simulink model "robot_forward"  (R2017a)
settings: Solver=FixedStepAuto  StartTime=0.0  StopTime=20  FixedStep=1e-3  RelTol=1e-3
settings Model: Creator=Jan  LastModifiedBy=Jan

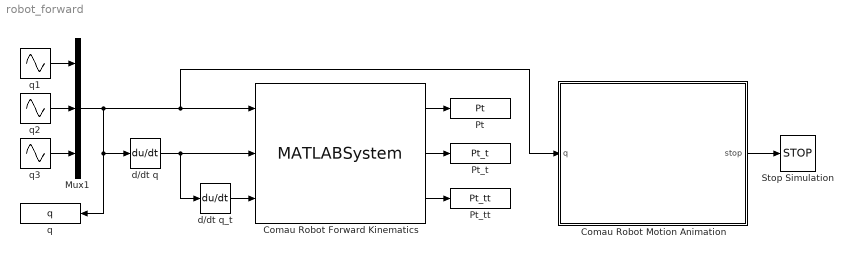
== system robot_forward ==
  Comau Robot Forward Kinematics : MATLABSystem  System=ComauRobotSystem  StringChoice=Forward Kinematics  SimulateUsing=Code generation
      mask Type: ComauRobotSystem
      mask Display:
      | disp('ComauRobotSystem');
      | port_label('input',1,'q');
      | port_label('input',2,'q_t');
      | port_label('input',3,'q_tt');
      | port_label('output',1,'Pt');
      | port_label('output',2,'Pt_t');
      | port_label('output',3,'Pt_tt');
  Comau Robot Motion Animation : MATLAB Function  TreatAsAtomicUnit=on  SystemSampleTime=0.1
  Mux1 : Mux  Inputs=3
  Pt : ToWorkspace  VariableName=Pt  SampleTime=-1
  Pt_t : ToWorkspace  VariableName=Pt_t  SampleTime=-1
  Pt_tt : ToWorkspace  VariableName=Pt_tt  SampleTime=-1
  Stop Simulation : Stop
  d/dt q : Derivative
  d/dt q_t : Derivative
  q : ToWorkspace  VariableName=q  SampleTime=-1
  q1 : Sin  Amplitude=30/180*pi*0  Bias=-15*pi/180*0  Frequency=2*pi*0.05  Phase=45/180*pi  SampleTime=0
  q2 : Sin  Amplitude=20/180*pi*0  Bias=-20*pi/180*0  Frequency=2*pi*0.1  Phase=90/180*pi  SampleTime=0
  q3 : Sin  Amplitude=15/180*pi*0  Bias=-pi/2*1 -55*pi/180*0  Frequency=2*pi*0.15  Phase=0/180*pi  SampleTime=0
  wires:
  Mux1/1 -> Comau Robot Motion Animation/1(q), Comau Robot Forward Kinematics/1, q/1, d/dt q/1
  q3/1 -> Mux1/3
  q2/1 -> Mux1/2
  d/dt q/1 -> d/dt q_t/1, Comau Robot Forward Kinematics/2
  q1/1 -> Mux1/1
  d/dt q_t/1 -> Comau Robot Forward Kinematics/3
  Comau Robot Motion Animation/1(stop) -> Stop Simulation/1
  Comau Robot Forward Kinematics/2 -> Pt_t/1
  Comau Robot Forward Kinematics/3 -> Pt_tt/1
  Comau Robot Forward Kinematics/1 -> Pt/1

== matlab function robot_forward/Comau Robot Motion Animation ==
  data: q input; stop output
function stop = SimulinkMotionPlot_Comau(q)
    % Creates a 3D-animation for the motion of the Comau Robot
    % Requires values for the Comau Robot joints
    
    % Persistent variables, to only be initialized once
    persistent h;           % Plot
    persistent Hr;          % Transformation Matrix
    stop = false;
    
    %% Initialization 
    % One time intitialization of plotting settings
    if isempty(h)
        % Plotting setup
        h = figure('Name','ComauRobot Animation');
        xlabel('x-axis')
        ylabel('y-axis')
        zlabel('z-axis')
        xlim([-2, 4])
        ylim([-2, 4])
        zlim([-1, 4])
        hold on;
        grid on;
        view(-20,20);
        
        % Relative Transformation to Robot Base
        Hr = eye(4);
    end
    
    %% Drawing
    if ishandle(h)
        cla;
        plot_robotpose(q, Hr);
        drawnow;
    end
    
    %% Destructor
    if ~ishandle(h)
        stop = true;
    end
end

%% Child functions

function plot_robotpose(q, Hr)
    % Plot the pose of the Comau Robot
    % This includes links and local coordinate systems

    % Inputs:
    % Hr : Transformation matrix of the robot base [4x4]
    % q  : Robot joints [3x1]
    
    % Static link lengths
    a1 = 0.350;
    a2 = 1.160;
    a3 = 0.250;
    d1 = 0.830;
    d4 = 1.4922;
    d6 = 0.210;
    dt = 0.567;
    L = d4 + d6 + dt;
    
    % Joint angles
    q1 = q(1);
    q2 = q(2);
    q3 = q(3);

    % Robot DH Table
    T1 = math3d.DH(-q1, d1, a1, pi/2);
    T2 = math3d.DH(pi/2 - q2, 0, a2, 0);
    T3 = math3d.DH(q3 + pi/2 + q2, 0, a3, pi/2);
    T4 = math3d.DH(pi, L, 0, 0);

    % Relative transformation
    Hr1 = Hr*T1;    % Robot base to joint q1 {r -> q1}
    Hr2 = Hr1*T2;   % Robot base to joint q2 {r -> q2}
    Hr3 = Hr2*T3;   % Robot base to joint q3 {r -> q2}
    Hr4 = Hr3*T4;   % Robot base to tool-point {r -> t}

    % Plot coordinate systems
    plot_coordinatesystem(Hr);      % Base
    plot_coordinatesystem(Hr1);     % Joint q1
    plot_coordinatesystem(Hr2);     % Joint q2
    plot_coordinatesystem(Hr3);     % Joint q3
    plot_coordinatesystem(Hr4);     % Tool-Point

    % Plot links
    plot_line(Hr(1:3,4), Hr1(1:3,4));	% Base to joint q1        
    plot_line(Hr1(1:3,4), Hr2(1:3,4));	% joint q1 to joint q2 
    plot_line(Hr2(1:3,4), Hr3(1:3,4));	% joint q2 to joint q3 
    plot_line(Hr3(1:3,4), Hr4(1:3,4));	% joint q3 to Tool-point
end

% Plot a line in 3D plots
function plot_line(p1, p2)
    % Inputs:
    %   p1  :   Point 1 [x1; y1; z1]
    %   p2  :   Point 2 [x2; y2; z2]

    % Pre-allocate
    line = zeros(2,3);
    
    line(1,:) = p1;
    line(2,:) = p2;

    X = line(:,1);
    Y = line(:,2);
    Z = line(:,3);

    plot3(X, Y, Z, 'k', 'LineWidth', 1)
end

% Plot the coordinate system in 3D plots
% with default rgb-colors to the related axis.
function plot_coordinatesystem(H)
    % Inputs:
    %   H       :   Transformation-matrix (size = 4x4)

    % Pre-allocate
    axis = zeros(2,3);

    % Rotation and Translation
    d = H(1:3,4);   % Translation vector
    R = H(1:3,1:3); % Rotation matrix

    % Axis colors
    colors = {'r', 'g', 'b'};

    % Length of each axis in csys
    csys_len = 0.5;

    % Plot all 3 axis
    % (Looping through plotting one axis at a time)
    for i = 1:3
        axis(1,:) = d;                      % csys origo [x0 y0 z0]
        axis(2,:) = d + R(:,i)*csys_len;    % end point of axis [x y z]

        X = axis(:,1);  % Vector of the x-component
        Y = axis(:,2);  % Vector of the y-component
        Z = axis(:,3);  % Vector of the z-component

        % Plot one of the axis with the related color
        plot3(X, Y, Z, colors{i}, 'LineWidth', 1)
    end
end
